simulink model "guid_stab_loop"  (R2021a)
settings: Solver=VariableStepAuto  StartTime=0.0  StopTime=10.0  RelTol=1e-3
settings Model: Creator=AutomZ2-RG02A02  LastModifiedBy=AutomZ2-RG02A02

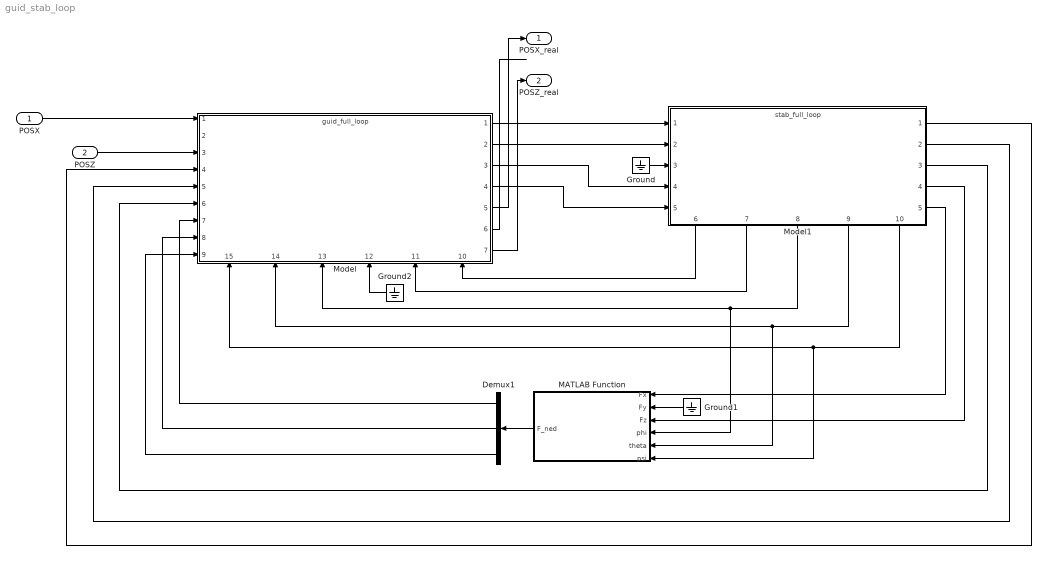
== system guid_stab_loop ==
  POSX : Inport
  POSZ : Inport  Port=2
  Demux1 : Demux  Outputs=3
  Ground : Ground
  Ground1 : Ground
  Ground2 : Ground
  MATLAB Function : MATLAB Function  TreatAsAtomicUnit=on
  Model : ModelReference  ModelNameDialog=guid_full_loop.slx  SimulationMode=Normal  ModelReferenceVersion=68
      settings: PortSchema="{\"entries\":[{\"content\":{\"sides\":[{\"content\":{\"connectorIds\":[\"In1\",\"In2\",\"In3\",\"In4\",\"In5\",\"In6\",\"In7\",\"In8\",\"In9\"]},\"type\":\"ConnectorPlacement.EquallySpacedRectSide\",\"uuid\":\"c7039e2d-4d2b-486c-8f74-6257b5d4cd10\"},{\"content\":{\"connectorIds\":[\"Out1\",\"Out2\",\"Out3\",\"Out4\",\"Out5\",\"Out6\",\"Out7\"],\"side\":\"RIGHT\"},\"type\":\"ConnectorPlacement.EquallySpacedRectSide\",\"uuid\":\"e0c80cde-7009-468d-bd8c-a0953f93fc9b\"},{\"content\":{\"connectorIds\":[],\"side\":\"TOP\"},\"type\":\"ConnectorPlacement.EquallySpacedRectSide\",\"uuid\":\"ae82e6b4-ee43-49bb-afd8-398584e62041\"},{\"content\":{\"connectorIds\":[\"In15\",\"In14\",\"In13\",\"In12\",\"In11\",\"In10\"],\"side\":\"BOTTOM\"},\"type\":\"ConnectorPlacement.EquallySpacedRectSide\",\"uuid\":\"bfc3b99b-31c9-45a2-8956-d202fb3b7ccc\"}]},\"type\":\"ConnectorPlacement.EquallySpacedConnector\",\"uuid\":\"314e09c4-e57e-4071-b616-dff2ef626096\"}],\"packageUris\":[\"http://schema.mathworks.com/mf0/Connector/R2020b\"],\"version\":\"1.0\"}"
  Model1 : ModelReference  ModelNameDialog=stab_full_loop.slx  SimulationMode=Normal  ModelReferenceVersion=60
      settings: PortSchema="{\"entries\":[{\"content\":{\"sides\":[{\"content\":{\"connectorIds\":[\"In1\",\"In2\",\"In3\",\"In4\",\"In5\"]},\"type\":\"ConnectorPlacement.EquallySpacedRectSide\",\"uuid\":\"6193f038-e962-4cc8-aa13-3f309e78671e\"},{\"content\":{\"connectorIds\":[\"Out1\",\"Out2\",\"Out3\",\"Out4\",\"Out5\"],\"side\":\"RIGHT\"},\"type\":\"ConnectorPlacement.EquallySpacedRectSide\",\"uuid\":\"4da1bbe6-45dc-40ed-8db5-843428d3d31a\"},{\"content\":{\"connectorIds\":[],\"side\":\"TOP\"},\"type\":\"ConnectorPlacement.EquallySpacedRectSide\",\"uuid\":\"7690dd6e-2966-44a8-8ce5-50dbef302b6f\"},{\"content\":{\"connectorIds\":[\"Out6\",\"Out7\",\"Out8\",\"Out9\",\"Out10\"],\"side\":\"BOTTOM\"},\"type\":\"ConnectorPlacement.EquallySpacedRectSide\",\"uuid\":\"16088e23-4634-4b26-b830-f671c4042f09\"}]},\"type\":\"ConnectorPlacement.EquallySpacedConnector\",\"uuid\":\"62b25bf1-d081-4997-9962-408723a8cd0a\"}],\"packageUris\":[\"http://schema.mathworks.com/mf0/Connector/R2020b\"],\"version\":\"1.0\"}"
  POSX_real : Outport
  POSZ_real : Outport  Port=2
  wires:
  Model/1 -> Model1/1
  Model/2 -> Model1/2
  Model/3 -> Model1/4
  Model/4 -> Model1/5
  Ground/1 -> Model1/3
  Model1/4 -> MATLAB Function/3(Fz)
  POSX/1 -> Model/1
  ? -> Model/2
  POSZ/1 -> Model/3
  Model1/1 -> Model/4
  Model1/2 -> Model/5
  Model1/3 -> Model/6
  Ground1/1 -> MATLAB Function/2(Fy)
  Demux1/1 -> Model/7
  Demux1/2 -> Model/8
  Demux1/3 -> Model/9
  Model1/7 -> Model/11
  Model1/8 -> Model/13, MATLAB Function/4(phi)
  Model1/9 -> Model/14, MATLAB Function/5(theta)
  Model1/10 -> Model/15, MATLAB Function/6(psi)
  Model1/5 -> MATLAB Function/1(Fx)
  MATLAB Function/1(F_ned) -> Demux1/1
  Model1/6 -> Model/10
  Ground2/1 -> Model/12
  Model/5 -> POSX_real/1
  Model/6 -> ?
  Model/7 -> POSZ_real/1

== matlab function guid_stab_loop/MATLAB Function ==
  data: Fx input; F_ned output; Fy input; Fz input; phi input; theta input; psi input
function F_ned = rotateBodyToNED(Fx, Fy, Fz, phi, theta, psi)

Fb = [Fx; Fy; Fz];

cphi = cos(phi);    sphi = sin(phi);
ctheta = cos(theta); stheta = sin(theta);
cpsi = cos(psi);    spsi = sin(psi);

R = [ cpsi*ctheta - spsi*sphi*stheta, -spsi*cphi,  cpsi*stheta + spsi*sphi*ctheta;
      spsi*ctheta + cpsi*sphi*stheta,  cpsi*cphi,  spsi*stheta - cpsi*sphi*ctheta;
     -cphi*stheta,                     sphi,       cphi*ctheta ];

F_ned = R * Fb;

end
